simulink model "rtwdemo_advisor1"  (Simulink 7.6)
settings: Solver=VariableStepDiscrete  SolverMode=SingleTasking  StartTime=0.0  StopTime=4  FixedStep=1  RelTol=1e-3  AbsTol=1e-6  SampleTimeConstraint=Specified
undefined symbols (not defined in the file or in its folder): DiscIntNeverNeededParam
libraries: simulink x1, rtwdemowidgets x1
Description:
  | Model Advisor -- Optimizing for Real-Time Deployment
settings Model: Creator=The MathWorks Inc.  CovMetricSettings=d  ExtModeTrigMode=oneshot  ExtModeArmWhenConnect=off  ExtModeAutoUpdateStatusClock=off
settings DataIOCC: LimitDataPoints=off  SaveFinalState=on  SaveOutput=off  SaveState=on  SignalLoggingName=sigsOut
settings OptimizationCC: InlineParams=on  InlineInvariantSignals=on  FoldNonRolledExpr=off  ZeroExternalMemoryAtStartup=off  ZeroInternalMemoryAtStartup=off  NoFixptDivByZeroProtection=on  EfficientFloat2IntCast=on  OptimizeModelRefInitCode=on
settings DebuggingCC: CheckExecutionContextPreStartOutputMsg=on  CheckExecutionContextRuntimeOutputMsg=on  SolverPrmCheckMsg=none  IntegerOverflowMsg=none  ParameterDowncastMsg=warning  ParameterOverflowMsg=warning  ParameterPrecisionLossMsg=none  UnconnectedInputMsg=none  UnconnectedOutputMsg=none  UnconnectedLineMsg=none  StrictBusMsg=ErrorOnBusTreatedAsVector
settings HardwareCC: ProdIntDivRoundTo=Zero  ProdEndianess=LittleEndian  ProdHWDeviceType=Generic->32-bit Embedded Processor  TargetHWDeviceType=Generic->32-bit Embedded Processor
settings SFSimCC: SimParseCustomCode=off
settings RTWCC: SystemTargetFile=ert.tlc  TemplateMakefile=ert_default_tmf  RTWVerbose=off  ProcessScript=ert_make_rtw_hook
settings CodeAppCC: GenerateComments=off  IgnoreCustomStorageClasses=off  IncHierarchyInIds=on  IncDataTypeInIds=on  SimulinkBlockComments=off  InlinedPrmAccess=Macros
settings ERTTargetCC: TargetFcnLib=ansi_tfl_tmw.mat  MultiwordLength=2048  GenerateSampleERTMain=on  MatFileLogging=on  SupportContinuousTime=on  ExtMode=on  ERTCustomFileTemplate=example_file_process.tlc  ConvertIfToSwitch=off

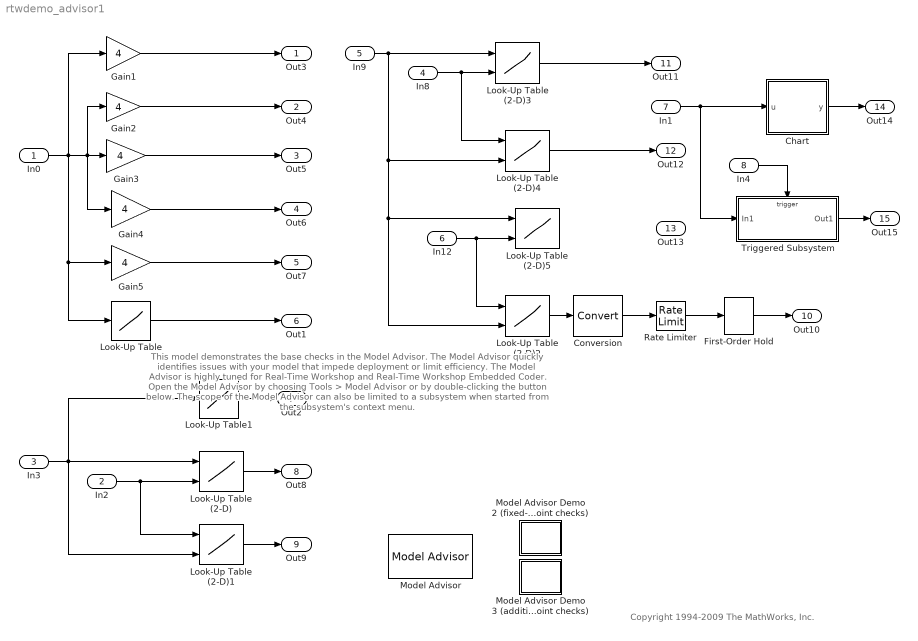
== system rtwdemo_advisor1 ==
  note: This model demonstrates the base checks in the Model Advisor.  The Model
      | Advisor quickly identifies issues with your model that impede deployment
      | or limit efficiency.  The Model Advisor is highly tuned for Real-Time Workshop
      | and Real-Time Workshop Embedded Coder.  Open the Model Advisor by
      | choosing Tools > Model Advisor or by double-clicking the button below.
      | The scope of the Model Advisor can also be limited to a subsystem when
      | started from the subsystem's context menu.
  note: Copyright 1994-2009 The MathWorks, Inc.
  In0 : Inport  OutDataTypeStr=uint8  Interpolate=off
  In2 : Inport  Port=2  OutDataTypeStr=uint32  Interpolate=off
  In3 : Inport  Port=3  OutDataTypeStr=uint32  Interpolate=off
  In8 : Inport  Port=4  OutDataTypeStr=uint16  Interpolate=off
  In9 : Inport  Port=5  OutDataTypeStr=uint16  Interpolate=off
  In12 : Inport  Port=6  OutDataTypeStr=uint16  Interpolate=off
  In1 : Inport  Port=7  OutDataTypeStr=double  PortDimensions=1  Interpolate=off
  In4 : Inport  Port=8  OutDataTypeStr=boolean  PortDimensions=1  Interpolate=off
  " Model Advisor Demo 2 (fixed-point checks)" : Subsystem
      settings: OpenFcn=rtwdemo_advisor2
      mask Display: disp('open')
  " Model Advisor Demo 3 (additional fixed-point checks)" : Subsystem
      settings: OpenFcn=rtwdemo_advisor3
      mask Display: disp('open')
  Chart : Stateflow chart  TreatAsAtomicUnit=on
  Conversion : DataTypeConversion  ConvertRealWorld=Stored Integer (SI)
  First-Order Hold : simulink/Discrete/First-Order Hold  SystemSampleTime=-1  Ts=1
  Gain1 : Gain  Gain=4  OutDataTypeStr=Inherit: Same as input  ParamDataTypeStr=Inherit: Same as input
  Gain2 : Gain  Gain=4  ParamDataTypeStr=fixdt(1,32,0)  SaturateOnIntegerOverflow=on  OutDataTypeStr=Inherit: Same as input
  Gain3 : Gain  Gain=4  ParamDataTypeStr=fixdt(1,32,0)  OutDataTypeStr=Inherit: Same as input
  Gain4 : Gain  Gain=4  ParamDataTypeStr=fixdt(1,32,0)  OutDataTypeStr=Inherit: Same as input
  Gain5 : Gain  Gain=4  ParamDataTypeStr=fixdt(1,32,0)  SaturateOnIntegerOverflow=on  OutDataTypeStr=Inherit: Same as input
  Look-Up Table : Lookup  InputValues=[0 1 3 7]  Table=[9 3 9 3]  LookUpMeth=Interpolation-Use End Values  OutDataTypeStr=int16  RndMeth=Nearest
  Look-Up Table (2-D) : Lookup2D  RowIndex=[1:3]  ColumnIndex=[1:3]  Table=[4 5 6;16 19 20;10 18 23]  LookUpMeth=Interpolation-Use End Values
  Look-Up Table (2-D)1 : Lookup2D  RowIndex=[0 2 5]  ColumnIndex=[1:3]  Table=[4 5 6;16 19 20;10 18 23]  LookUpMeth=Interpolation-Use End Values
  Look-Up Table (2-D)2 : Lookup2D  RowIndex=[1:3]  ColumnIndex=[1 2 7]  Table=[4 5 6;16 19 20;10 18 23]  LookUpMeth=Interpolation-Use End Values  OutDataTypeStr=uint32
  Look-Up Table (2-D)3 : Lookup2D  RowIndex=[1:3]  ColumnIndex=[1:3]  Table=[4 5 6;16 19 20;10 18 23]  LookUpMeth=Interpolation-Use End Values
  Look-Up Table (2-D)4 : Lookup2D  RowIndex=[1:3]  ColumnIndex=[1 2 3 4 5]  Table=ones(3,5)  LookUpMeth=Interpolation-Use End Values  OutDataTypeStr=uint16
  Look-Up Table (2-D)5 : Lookup2D  RowIndex=[6 7 8 9 10]  ColumnIndex=[1:3]  Table=ones(3,5).'  LookUpMeth=Interpolation-Use End Values  OutDataTypeStr=int16
  Look-Up Table1 : Lookup  InputValues=[20 21 22 23 24]  Table=[9 3 9 3 9]  LookUpMeth=Interpolation-Use End Values  OutDataTypeStr=uint16
  Model Advisor : rtwdemowidgets/Model Advisor  SystemSampleTime=-1  attrib_overrides={}
  Rate Limiter : RateLimiter
  Triggered Subsystem : Subsystem  TreatAsAtomicUnit=on
  Out3 : Outport
  Out4 : Outport  Port=2
  Out5 : Outport  Port=3
  Out6 : Outport  Port=4
  Out7 : Outport  Port=5
  Out1 : Outport  Port=6
  Out2 : Outport  Port=7
  Out8 : Outport  Port=8
  Out9 : Outport  Port=9
  Out10 : Outport  Port=10
  Out11 : Outport  Port=11
  Out12 : Outport  Port=12
  Out13 : Outport  Port=13
  Out14 : Outport  Port=14
  Out15 : Outport  Port=15
  wires:
  Gain1/1 -> Out3/1
  Gain2/1 -> Out4/1
  Gain3/1 -> Out5/1
  Gain4/1 -> Out6/1
  Gain5/1 -> Out7/1
  Look-Up Table/1 -> Out1/1
  Look-Up Table1/1 -> Out2/1
  In2/1 -> Look-Up Table (2-D)/2, Look-Up Table (2-D)1/1
  Look-Up Table (2-D)/1 -> Out8/1
  In3/1 -> Look-Up Table (2-D)/1, Look-Up Table (2-D)1/2, Look-Up Table1/1
  Look-Up Table (2-D)1/1 -> Out9/1
  Look-Up Table (2-D)2/1 -> Conversion/1
  In8/1 -> Look-Up Table (2-D)4/1, Look-Up Table (2-D)3/2
  Look-Up Table (2-D)3/1 -> Out11/1
  In9/1 -> Look-Up Table (2-D)4/2, Look-Up Table (2-D)5/1, Look-Up Table (2-D)2/2, Look-Up Table (2-D)3/1
  Look-Up Table (2-D)4/1 -> Out12/1
  In12/1 -> Look-Up Table (2-D)5/2, Look-Up Table (2-D)2/1
  Rate Limiter/1 -> First-Order Hold/1
  Conversion/1 -> Rate Limiter/1
  First-Order Hold/1 -> Out10/1
  In0/1 -> Gain3/1, Gain4/1, Gain2/1, Gain1/1, Gain5/1, Look-Up Table/1
  In1/1 -> Chart/1(u), Triggered Subsystem/1(In1)
  Chart/1(y) -> Out14/1
  Triggered Subsystem/1(Out1) -> Out15/1
  In4/1 -> Triggered Subsystem/Trigger

== system rtwdemo_advisor1/ Model Advisor Demo 2 (fixed-point checks) ==

== system rtwdemo_advisor1/ Model Advisor Demo 3 (additional fixed-point checks) ==

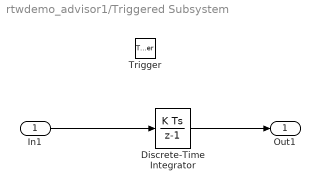
== system rtwdemo_advisor1/Triggered Subsystem ==
  In1 : Inport
  Trigger : TriggerPort
  Discrete-Time Integrator : DiscreteIntegrator  InitialConditionMode=State only (most efficient)  SampleTime=-1  ICPrevOutput=DiscIntNeverNeededParam  ICPrevScaledInput=DiscIntNeverNeededParam
  Out1 : Outport  InitialOutput=0
  wires:
  In1/1 -> Discrete-Time Integrator/1
  Discrete-Time Integrator/1 -> Out1/1

== stateflow chart Chart ==
  state B
  state A
  A -> B : {y=u*2;}
  (default) -> A
  data: u input int32; y output int32
